simulink model "Longitudinal_Motion_JoystickO_Auto_Pilot"  (R2018b)
settings: Solver=ode4  StartTime=0.0  StopTime=30  FixedStep=0.01  RelTol=1e-3
values from neighbouring files (symbols this model uses):
  m = max(dataTrain)    [CodeShortPeriod.m]
undefined symbols (not defined in the file or in its folder): alpha0, c, CL_alpha, Cm_alpha, Cm_alpha_dot, Cm_delta, Cm_q, Cx0, ft, G, Iy, K, Pmax, s, S, Vmax
libraries: aerolibconvert2 x3, simulink x1, aerolibatmos2 x1, vrlib x1, simulink_extras x1, sldrtlib x1
settings Model: Creator=aiham  LastModifiedBy=aiham

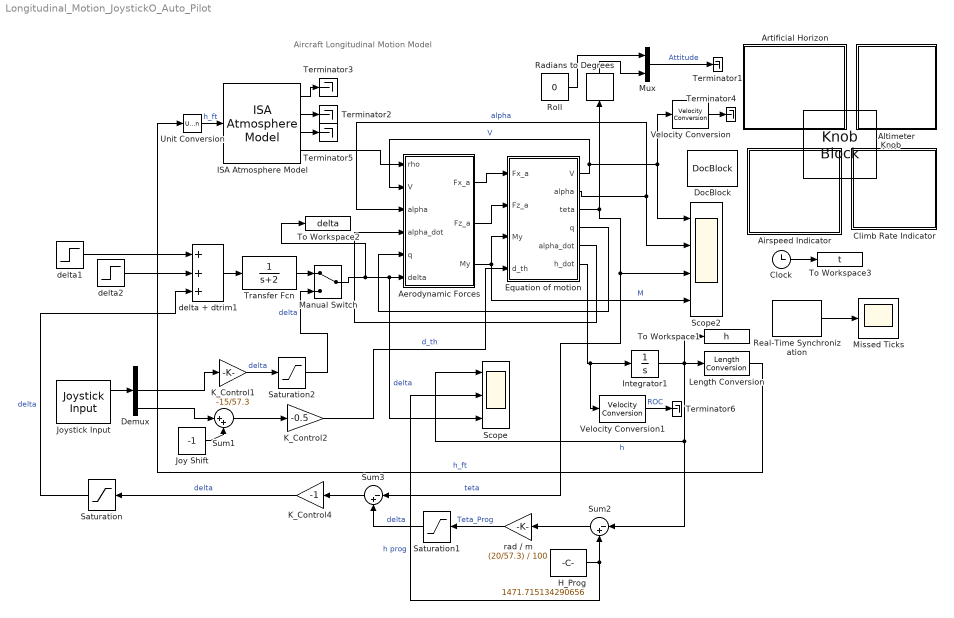
== system Longitudinal_Motion_JoystickO_Auto_Pilot ==
  note: Aircraft Longitudinal Motion Model
  Aerodynamic Forces : Subsystem
  Airspeed Indicator : Subsystem  DialogController=aeroblksHMICreateDDGDialog  IsWebBlock=on  mask(MWDashboardBlock){webBlockId=39b6216f-d8bc-451e-94a0-620830d44ccc, webBlockType=airspeedindicator, ShowInLibBrowser=on, ShowInitialText=on, HMISrcModelName=Longitudinal_Motion_Joystick}
      mask prompts: webBlockId "WebBlock Id"; webBlockType "WebBlock Type"; HMISrcModelName "Source Model"
      mask help: aeroblksHMI:aeroblkhmi:AirspeedIndicatorDialogDesc
      mask Help: eval('asbhmihelp(''airspeedindicator'')');
      mask Display:
      | if strcmp(get_param(bdroot(gcb),'BlockDiagramType'), 'library')
      |  image([(matlabroot) '/toolbox/aeroblks/aeroblks/hmi/icons/AirspeedIndicatorIcon.svg'])
      | end
  Altimeter : Subsystem  DialogController=aeroblksHMICreateDDGDialog  IsWebBlock=on  mask(MWDashboardBlock){webBlockId=6156dfbe-d862-4082-9787-1997ae738bde, webBlockType=altimeter, ShowInLibBrowser=on, ShowInitialText=on, HMISrcModelName=Longitudinal_Motion_Joystick}
      mask prompts: webBlockId "WebBlock Id"; webBlockType "WebBlock Type"; HMISrcModelName "Source Model"
      mask help: aeroblksHMI:aeroblkhmi:AltimeterDialogDesc
      mask Help: eval('asbhmihelp(''altimeter'')');
      mask Display:
      | if strcmp(get_param(bdroot(gcb),'BlockDiagramType'), 'library')
      |  image([(matlabroot) '/toolbox/aeroblks/aeroblks/hmi/icons/AltimeterIcon.svg'])
      | end
  Artificial Horizon : Subsystem  DialogController=aeroblksHMICreateDDGDialog  IsWebBlock=on  mask(MWDashboardBlock){webBlockId=ab1fbaf0-e3e3-44e6-8da3-0beb0e23903c, webBlockType=artificialhorizon, ShowInLibBrowser=on, ShowInitialText=on, HMISrcModelName=Longitudinal_Motion_Joystick}
      mask prompts: webBlockId "WebBlock Id"; webBlockType "WebBlock Type"; HMISrcModelName "Source Model"
      mask help: aeroblksHMI:aeroblkhmi:ArtificialHorizonDialogDesc
      mask Help: eval('asbhmihelp(''artificialhorizon'')');
      mask Display:
      | if strcmp(get_param(bdroot(gcb),'BlockDiagramType'), 'library')
      |  image([(matlabroot) '/toolbox/aeroblks/aeroblks/hmi/icons/ArtificialHorizonIcon.svg'])
      | end
  Climb Rate Indicator : Subsystem  DialogController=aeroblksHMICreateDDGDialog  IsWebBlock=on  mask(MWDashboardBlock){webBlockId=113527b1-61e3-4069-bf92-54d9ccf41337, webBlockType=climbindicator, ShowInLibBrowser=on, ShowInitialText=on, HMISrcModelName=Longitudinal_Motion_Joystick}
      mask prompts: webBlockId "WebBlock Id"; webBlockType "WebBlock Type"; HMISrcModelName "Source Model"
      mask help: aeroblksHMI:aeroblkhmi:ClimbIndicatorDialogDesc
      mask Help: eval('asbhmihelp(''climbindicator'')');
      mask Display:
      | if strcmp(get_param(bdroot(gcb),'BlockDiagramType'), 'library')
      |  image([(matlabroot) '/toolbox/aeroblks/aeroblks/hmi/icons/ClimbIndicatorIcon.svg'])
      | end
  Clock : Clock
  Demux : Demux  Outputs=3
  DocBlock : simulink/Model-Wide Utilities/DocBlock  DocumentType=Text
      content=|
      | % Type your documentation here
      | m = 900;      % kg
      | G = m * 9.81; % N
      |
      | Iy = 2900;    % kg m2
      | S = 12;       % m2
      | c = 1.5;      % m
      | Cx0 = 0.03;
      | K = 0.072; %%%%% Check
      | alpha0 = -4   / 57.3  % rad
      | CL_alpha = 4.6;
      |
      | Cm_alpha = -0.89
      | Cm_alpha_dot = -5.2
      | Cm_q = -12.4
      | Cm_delta = -1.0;
      |
      | Vmax = 260 / 3.6;
      | Pmax = 400 * 9.81;   % N
      | V0 = 150 / 3.6;    % m/s
      | teta0 = 0;  % rad
      | gamma0 = 0; % rad
  Equation of motion : Subsystem
  H_Prog : Constant  Value=1471.715134290656
  ISA Atmosphere Model : aerolibatmos2/ISA Atmosphere Model  custom=off  g=9.80665  gamma=1.4  R=287.0531  L=0.0065  h_trop=11000  h_strat=20000  rho0=1.225  P0=101325  T0=288.15  h0=0
      settings: SourceProductName=Aerospace Blockset
  Integrator1 : Integrator  InitialCondition=1000
  Joy Shift : Constant  Value=-1
  Joystick Input : vrlib/Joystick Input  joyid=1  adjustports=on  forcefeed=off
      settings: SourceProductBaseCode=VR
  K_Control1 : Gain  Gain=-15/57.3
  K_Control2 : Gain  Gain=-0.5
  K_Control4 : Gain  Gain=-1
  Knob : KnobBlock  WebBlockId=305  ScaleMin=500  ScaleMax=2500  TickInterval=500
  Length Conversion : aerolibconvert2/Length Conversion  IU=m  OU=ft
  Manual Switch : ManualSwitch
  Missed Ticks : Scope
  Mux : Mux  Inputs=2
  Radians to Degrees : simulink_extras/Transformations/Radians to Degrees
  Real-Time Synchronization : sldrtlib/Real-Time Synchronization  SampleTime=0.01  MaxMissedTicks=100  ShowMissedTicks=on  YieldWhenWaiting=off
  Roll : Constant  Value=0
  Saturation : Saturate  UpperLimit=25 /57.3  LowerLimit=-25 /57.3
  Saturation1 : Saturate  UpperLimit=10 /57.3  LowerLimit=-15 /57.3
  Saturation2 : Saturate  UpperLimit=30 /57.3  LowerLimit=-30 /57.3
  Scope : Scope  NumInputPorts=3
  Scope2 : Scope  NumInputPorts=4
  Sum1 : Sum  Inputs=|++
  Sum2 : Sum  Inputs=|-+
  Sum3 : Sum  Inputs=|-+
  Terminator{1..6} (6 alike) : Terminator
  To Workspace1 : ToWorkspace  VariableName=h  SaveFormat=Timeseries  SampleTime=0.05
  To Workspace2 : ToWorkspace  VariableName=delta  SaveFormat=Timeseries  SampleTime=0.05
  To Workspace3 : ToWorkspace  VariableName=t  SaveFormat=Timeseries  SampleTime=0.05
  Transfer Fcn : TransferFcn  Denominator="[1  2]"
  Unit Conversion : UnitConversion
  Velocity Conversion : aerolibconvert2/Velocity Conversion  IU=m/s  OU=kts
  Velocity Conversion1 : aerolibconvert2/Velocity Conversion  IU=m/s  OU=ft/min
  delta + dtrim1 : Sum  Inputs=+++
  delta1 : Step  Time=5  After=- (5 / 57.3)  SampleTime=0
  delta2 : Step  Time=5.5  After=(5 / 57.3)  SampleTime=0
  rad / m : Gain  Gain=(20/57.3) / 100
  wires:
  Aerodynamic Forces/3(My) -> Equation of motion/3(My), Scope2/4  "M"
  Aerodynamic Forces/1(Fx_a) -> Equation of motion/1(Fx_a)
  Aerodynamic Forces/2(Fz_a) -> Equation of motion/2(Fz_a)
  ISA Atmosphere Model/4 -> Aerodynamic Forces/1(rho)
  ISA Atmosphere Model/1 -> Terminator3/1
  ISA Atmosphere Model/2 -> Terminator2/1
  ISA Atmosphere Model/3 -> Terminator5/1
  Equation of motion/1(V) -> Velocity Conversion/1, Scope2/1, Aerodynamic Forces/2(V)  "V"
  Equation of motion/2(alpha) -> Aerodynamic Forces/3(alpha), Scope2/2  "alpha"
  Equation of motion/4(q) -> Aerodynamic Forces/5(q)
  Equation of motion/3(teta) -> Sum3/1, Scope2/3, Radians to Degrees/1  "teta"
  Roll/1 -> Mux/1
  Mux/1 -> Terminator1/1  "Attitude"
  Radians to Degrees/1 -> Mux/2
  Equation of motion/5(alpha_dot) -> Aerodynamic Forces/4(alpha_dot)
  Saturation/1 -> delta + dtrim1/3  "delta"
  Manual Switch/1 -> To Workspace2/1, Scope/3, Aerodynamic Forces/6(delta)  "delta"
  Demux/2 -> K_Control1/1
  Real-Time Synchronization/1 -> Missed Ticks/1
  Equation of motion/6(h_dot) -> Velocity Conversion1/1, Integrator1/1
  Integrator1/1 -> To Workspace1/1, Scope/1, Sum2/1, Length Conversion/1  "h"
  Length Conversion/1 -> Unit Conversion/1  "h_ft"
  Velocity Conversion/1 -> Terminator4/1
  Unit Conversion/1 -> ISA Atmosphere Model/1  "h_ft"
  K_Control2/1 -> Equation of motion/4(d_th)  "d_th"
  Demux/3 -> Sum1/1
  Joy Shift/1 -> Sum1/2
  Sum1/1 -> K_Control2/1
  H_Prog/1 -> Scope/2, Sum2/2  "h prog"
  Sum2/1 -> rad / m/1
  rad / m/1 -> Saturation1/1  "Teta_Prog"
  Sum3/1 -> K_Control4/1
  K_Control4/1 -> Saturation/1  "delta"
  Saturation1/1 -> Sum3/2  "delta"
  delta2/1 -> delta + dtrim1/2
  delta1/1 -> delta + dtrim1/1
  delta + dtrim1/1 -> Transfer Fcn/1
  Transfer Fcn/1 -> Manual Switch/1
  Clock/1 -> To Workspace3/1
  Velocity Conversion1/1 -> Terminator6/1  "ROC"
  Joystick Input/1 -> Demux/1
  K_Control1/1 -> Saturation2/1  "delta"
  Saturation2/1 -> Manual Switch/2  "delta"

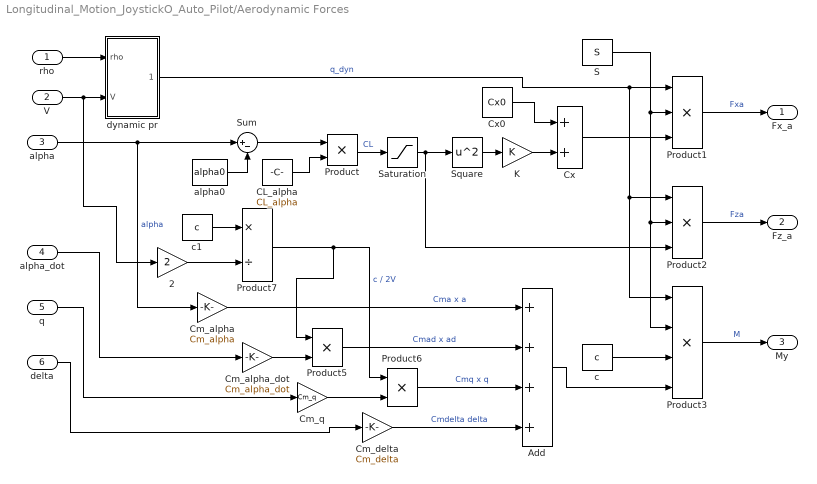
== system Longitudinal_Motion_JoystickO_Auto_Pilot/Aerodynamic Forces ==
  rho : Inport
  V : Inport  Port=2
  alpha : Inport  Port=3
  alpha_dot : Inport  Port=4
  q : Inport  Port=5
  delta : Inport  Port=6
  2 : Gain  Gain=2
  Add : Sum  Inputs=++++
  CL_alpha : Constant  Value=CL_alpha
  Cm_alpha : Gain  Gain=Cm_alpha
  Cm_alpha_dot : Gain  Gain=Cm_alpha_dot
  Cm_delta : Gain  Gain=Cm_delta
  Cm_q : Gain  Gain=Cm_q
  Cx : Sum
  Cx0 : Constant  Value=Cx0
  K : Gain  Gain=K
  Product : Product
  Product1 : Product  Inputs=3
  Product2 : Product  Inputs=3
  Product3 : Product  Inputs=4
  Product5 : Product
  Product6 : Product
  Product7 : Product  Inputs=*/
  S : Constant  Value=S
  Saturation : Saturate  UpperLimit=1.4  LowerLimit=-1.0
  Square : Math  Operator=square  SaturateOnIntegerOverflow=on
  Sum : Sum  Inputs=|+-
  alpha0 : Constant  Value=alpha0
  c : Constant  Value=c
  c1 : Constant  Value=c
  dynamic pr : Subsystem
  Fx_a : Outport
  Fz_a : Outport  Port=2
  My : Outport  Port=3
  wires:
  rho/1 -> dynamic pr/1(rho)
  Cx0/1 -> Cx/1
  CL_alpha/1 -> Product/2
  alpha0/1 -> Sum/2
  Sum/1 -> Product/1
  Product/1 -> Saturation/1  "CL"
  K/1 -> Cx/2
  Square/1 -> K/1
  Cx/1 -> Product1/3
  dynamic pr/1(q_dyn) -> Product1/1, Product2/1, Product3/1  "q_dyn"
  S/1 -> Product1/2, Product2/2, Product3/2
  alpha/1 -> Sum/1, Cm_alpha/1  "alpha"
  V/1 -> 2/1, dynamic pr/2(V)
  alpha_dot/1 -> Cm_alpha_dot/1
  q/1 -> Cm_q/1
  Cm_delta/1 -> Add/4  "Cmdelta delta"
  delta/1 -> Cm_delta/1
  c/1 -> Product3/3
  Product3/1 -> My/1  "M"
  Product5/1 -> Add/2  "Cmad x ad"
  Cm_alpha_dot/1 -> Product5/2
  Cm_q/1 -> Product6/2
  Product6/1 -> Add/3  "Cmq x q"
  Product7/1 -> Product5/1, Product6/1  "c / 2V"
  c1/1 -> Product7/1
  2/1 -> Product7/2
  Product1/1 -> Fx_a/1  "Fxa"
  Product2/1 -> Fz_a/1  "Fza"
  Cm_alpha/1 -> Add/1  "Cma x a"
  Add/1 -> Product3/4
  Saturation/1 -> Product2/3, Square/1

== system Longitudinal_Motion_JoystickO_Auto_Pilot/Airspeed Indicator ==

== system Longitudinal_Motion_JoystickO_Auto_Pilot/Altimeter ==

== system Longitudinal_Motion_JoystickO_Auto_Pilot/Artificial Horizon ==

== system Longitudinal_Motion_JoystickO_Auto_Pilot/Climb Rate Indicator ==

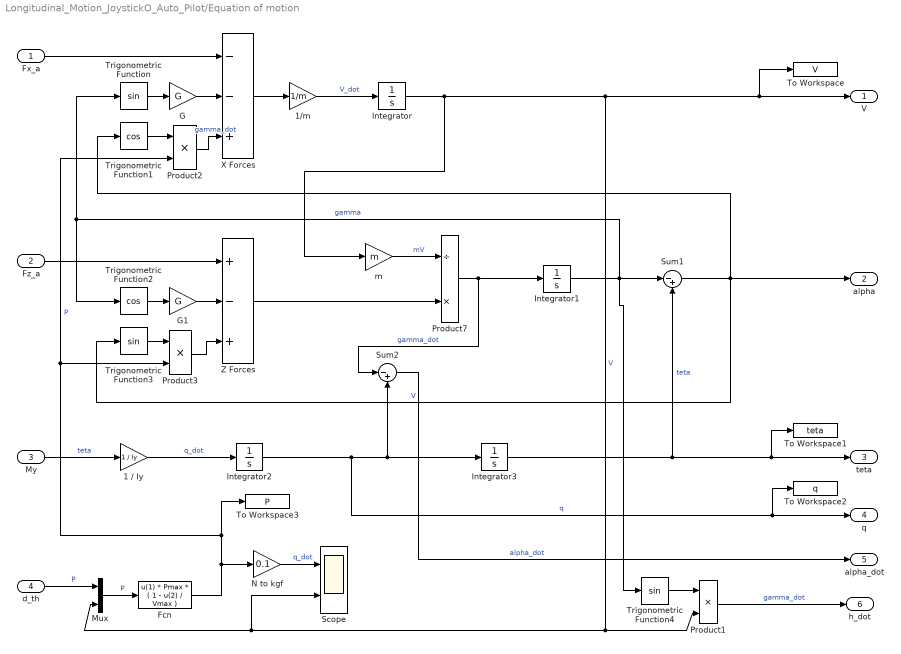
== system Longitudinal_Motion_JoystickO_Auto_Pilot/Equation of motion ==
  Fx_a : Inport
  Fz_a : Inport  Port=2
  My : Inport  Port=3
  d_th : Inport  Port=4
  1 / Iy : Gain  Gain=1 / Iy
  1/m : Gain  Gain=1/m
  Fcn : Fcn  Expr="u(1) * Pmax * ( 1  -  u(2) / Vmax )"
  G : Gain  Gain=G
  G1 : Gain  Gain=G
  Integrator : Integrator  InitialCondition=200 / 3.6
  Integrator1 : Integrator  InitialCondition=0 / 57.3
  Integrator2 : Integrator
  Integrator3 : Integrator  InitialCondition="0  / 57.3"
  Mux : Mux  Inputs=2
  N to kgf : Gain  Gain=0.1
  Product1 : Product  Inputs=**
  Product2 : Product  Inputs=**
  Product3 : Product  Inputs=**
  Product7 : Product  Inputs=/*
  Scope : Scope  NumInputPorts=2
  Sum1 : Sum  Inputs=|-+
  Sum2 : Sum  Inputs=|-+
  To Workspace : ToWorkspace  VariableName=V  SaveFormat=Timeseries  SampleTime=0.05
  To Workspace1 : ToWorkspace  VariableName=teta  SaveFormat=Timeseries  SampleTime=0.05
  To Workspace2 : ToWorkspace  VariableName=q  SaveFormat=Timeseries  SampleTime=0.05
  To Workspace3 : ToWorkspace  VariableName=P  SaveFormat=Timeseries  SampleTime=0.05
  Trigonometric Function : Trigonometry
  Trigonometric Function1 : Trigonometry  Operator=cos
  Trigonometric Function2 : Trigonometry  Operator=cos
  Trigonometric Function3 : Trigonometry
  Trigonometric Function4 : Trigonometry
  X Forces : Sum  Inputs=--+
  Z Forces : Sum  Inputs=+-+
  m : Gain  Gain=m
  V : Outport
  alpha : Outport  Port=2
  teta : Outport  Port=3
  q : Outport  Port=4
  alpha_dot : Outport  Port=5
  h_dot : Outport  Port=6
  wires:
  Integrator/1 -> m/1, To Workspace/1, V/1, Product1/2, Scope/2, Mux/2  "V"
  1/m/1 -> Integrator/1  "V_dot"
  Product7/1 -> Sum2/1, Integrator1/1  "gamma_dot"
  Trigonometric Function/1 -> G/1
  G/1 -> X Forces/2
  X Forces/1 -> 1/m/1
  Fx_a/1 -> X Forces/1
  Integrator1/1 -> Trigonometric Function2/1, Trigonometric Function/1, Trigonometric Function4/1, Sum1/1  "gamma"
  Integrator3/1 -> To Workspace1/1, teta/1, Sum1/2  "teta"
  Fz_a/1 -> Z Forces/1
  Trigonometric Function2/1 -> G1/1
  G1/1 -> Z Forces/2
  Trigonometric Function1/1 -> Product2/1
  m/1 -> Product7/1  "mV"
  Trigonometric Function3/1 -> Product3/1
  Product3/1 -> Z Forces/3
  My/1 -> 1 / Iy/1  "teta"
  1 / Iy/1 -> Integrator2/1  "q_dot"
  Integrator2/1 -> To Workspace2/1, q/1, Sum2/2, Integrator3/1  "q"
  Sum2/1 -> alpha_dot/1  "alpha_dot"
  Z Forces/1 -> Product7/2
  Product1/1 -> h_dot/1  "gamma_dot"
  Trigonometric Function4/1 -> Product1/1
  Fcn/1 -> N to kgf/1, To Workspace3/1, Product3/2, Product2/2  "P"
  Product2/1 -> X Forces/3  "gamma_dot"
  d_th/1 -> Mux/1  "P"
  Mux/1 -> Fcn/1  "P"
  N to kgf/1 -> Scope/1  "q_dot"
  Sum1/1 -> Trigonometric Function1/1, alpha/1, Trigonometric Function3/1  "V"

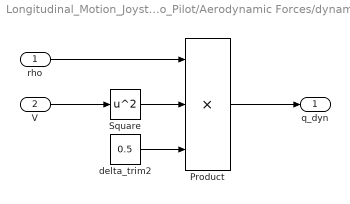
== system Longitudinal_Motion_JoystickO_Auto_Pilot/Aerodynamic Forces/dynamic pr ==
  rho : Inport
  V : Inport  Port=2
  Product : Product  Inputs=3
  Square : Math  Operator=square  SaturateOnIntegerOverflow=on
  delta_trim2 : Constant  Value=0.5
  q_dyn : Outport
  wires:
  rho/1 -> Product/1
  delta_trim2/1 -> Product/3
  V/1 -> Square/1
  Product/1 -> q_dyn/1
  Square/1 -> Product/2
